simulink model "verify_Thermal_Capacity_mdl"  (R2016b)
settings: Solver=ode45  StartTime=0.0  StopTime=4*3600  MaxStep=100  RelTol=1e-3  EnableMultiTasking=on
libraries: simulink x1, carnot x1
settings Model: Creator=drhf  LastModifiedBy=srrt
settings DataIOCC: LimitDataPoints=on  SaveFormat=Array  SignalLoggingSaveFormat=ModelDataLogs
settings OptimizationCC: ExpressionDepthLimit=2147483647  LifeSpan=inf
settings DebuggingCC: UnderspecifiedInitializationDetection=Classic  MergeDetectMultiDrivingBlocksExec=none  SolverPrmCheckMsg=warning  FcnCallInpInsideContextMsg=warning  StateNameClashWarn=warning  SFUnexpectedBacktrackingDiag=warning  SFNoUnconditionalDefaultTransitionDiag=warning  SFExecutionAtInitializationDiag=none
settings HardwareCC: ProdBitPerPointer=32  ProdBitPerSizeT=32  ProdBitPerPtrDiffT=32  ProdLargestAtomicFloat=None  ProdIntDivRoundTo=Undefined  ProdEndianess=Unspecified  ProdWordSize=32  ProdHWDeviceType=32-bit Generic
settings ModelReferenceCC: PropagateSignalLabelsOutOfModel=off
settings GRTTargetCC: TargetLangStandard=C89/C90 (ANSI)  GeneratePreprocessorConditionals=Disable all  CombineOutputUpdateFcns=off  GRTInterface=on
settings ConfigComp: CovMetricSettings=dw  CovHtmlReporting=on  CovSaveCumulativeToWorkspaceVar=on  CovSaveSingleToWorkspaceVar=on  CovExternalEMLEnable=off

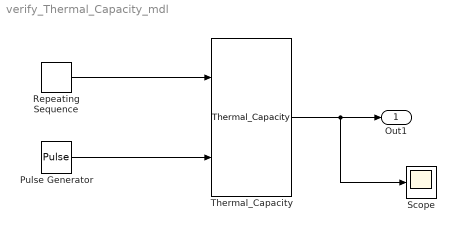
== system verify_Thermal_Capacity_mdl ==
  Pulse Generator : DiscretePulseGenerator  PulseType=Time based  Amplitude=100/3600  Period=2*3600  PulseWidth=50
  Repeating Sequence : simulink/Sources/Repeating Sequence  rep_seq_t=[0 2 2.1 4]*3600  rep_seq_y=[35 35 45 45]
  Scope : Scope
  Thermal_Capacity : carnot/Basic/Thermal_Models/Thermal_Capacity  UA=1  mcp=4182*10  Tamb=20  cp_approx=4000
  Out1 : Outport
  wires:
  Thermal_Capacity/1 -> Scope/1, Out1/1
  Pulse Generator/1 -> Thermal_Capacity/2
  Repeating Sequence/1 -> Thermal_Capacity/1
